simulink model "mux16to1"  (R2020a)
settings: Solver=VariableStepAuto  StartTime=0.0  StopTime=10.0  RelTol=1e-3
settings Model: Creator=kishan  LastModifiedBy=kishan

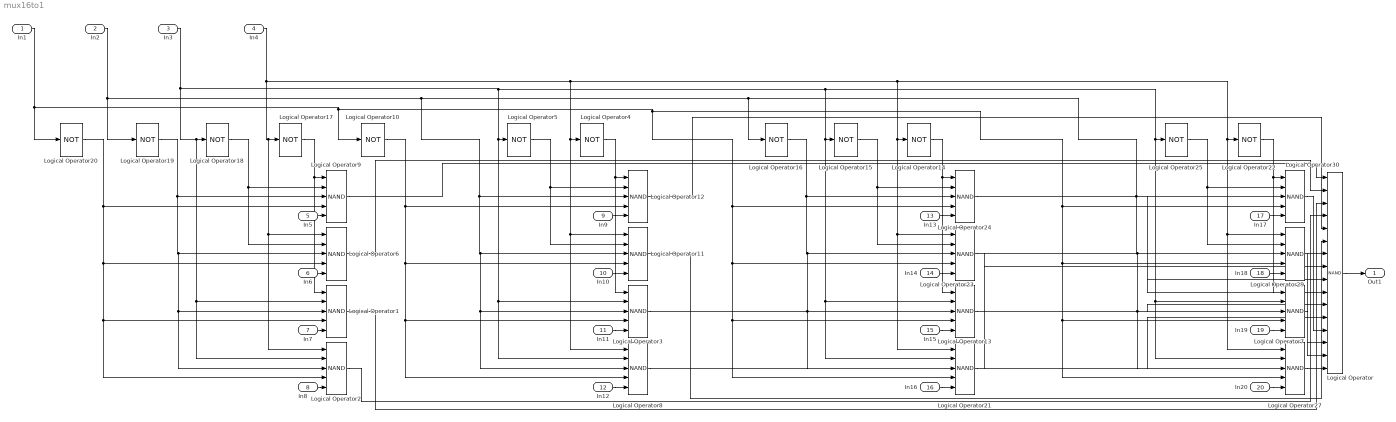
== system mux16to1 ==
  In1 : Inport
  In2 : Inport  Port=2
  In3 : Inport  Port=3
  In4 : Inport  Port=4
  In5 : Inport  Port=5
  In6 : Inport  Port=6
  In7 : Inport  Port=7
  In8 : Inport  Port=8
  In9 : Inport  Port=9
  In10 : Inport  Port=10
  In11 : Inport  Port=11
  In12 : Inport  Port=12
  In13 : Inport  Port=13
  In14 : Inport  Port=14
  In15 : Inport  Port=15
  In16 : Inport  Port=16
  In17 : Inport  Port=17
  In18 : Inport  Port=18
  In19 : Inport  Port=19
  In20 : Inport  Port=20
  Logical Operator : Logic  Operator=NAND  Inputs=16  AllPortsSameDT=off  OutDataTypeStr=boolean
  Logical Operator{1..3,6..9,11..13,21,23..24,27,29..30} (16 alike) : Logic  Operator=NAND  Inputs=5  AllPortsSameDT=off  OutDataTypeStr=boolean
  Logical Operator{4..5,10,14..20,22,25} (12 alike) : Logic  Operator=NOT  AllPortsSameDT=off  OutDataTypeStr=boolean
  Out1 : Outport
  wires:
  Logical Operator17/1 -> Logical Operator1/1, Logical Operator9/1
  Logical Operator18/1 -> Logical Operator6/2, Logical Operator9/2
  Logical Operator19/1 -> Logical Operator2/3, Logical Operator1/3, Logical Operator6/3, Logical Operator9/3
  Logical Operator20/1 -> Logical Operator2/4, Logical Operator1/4, Logical Operator6/4, Logical Operator9/4
  Logical Operator5/1 -> Logical Operator11/2, Logical Operator12/2
  Logical Operator4/1 -> Logical Operator3/1, Logical Operator12/1
  Logical Operator10/1 -> Logical Operator8/4, Logical Operator3/4, Logical Operator11/4, Logical Operator12/4
  Logical Operator15/1 -> Logical Operator23/2, Logical Operator24/2
  Logical Operator16/1 -> Logical Operator21/3, Logical Operator13/3, Logical Operator23/3, Logical Operator24/3
  Logical Operator14/1 -> Logical Operator13/1, Logical Operator24/1
  In4/1 -> Logical Operator27/1, Logical Operator29/1, Logical Operator22/1, Logical Operator21/1, Logical Operator23/1, Logical Operator14/1, Logical Operator8/1, Logical Operator11/1, Logical Operator4/1, Logical Operator2/1, Logical Operator6/1, Logical Operator17/1
  In3/1 -> Logical Operator21/2, Logical Operator13/2, Logical Operator15/1, Logical Operator27/2, Logical Operator7/2, Logical Operator25/1, Logical Operator8/2, Logical Operator3/2, Logical Operator5/1, Logical Operator2/2, Logical Operator1/2, Logical Operator18/1
  Logical Operator25/1 -> Logical Operator29/2, Logical Operator30/2
  In2/1 -> Logical Operator8/3, Logical Operator3/3, Logical Operator11/3, Logical Operator12/3, Logical Operator27/3, Logical Operator7/3, Logical Operator29/3, Logical Operator30/3, Logical Operator16/1, Logical Operator19/1
  Logical Operator22/1 -> Logical Operator7/1, Logical Operator30/1
  In1/1 -> Logical Operator27/4, Logical Operator7/4, Logical Operator29/4, Logical Operator30/4, Logical Operator21/4, Logical Operator13/4, Logical Operator23/4, Logical Operator24/4, Logical Operator10/1, Logical Operator20/1
  Logical Operator9/1 -> Logical Operator/1
  Logical Operator6/1 -> Logical Operator/2
  Logical Operator1/1 -> Logical Operator/3
  Logical Operator2/1 -> Logical Operator/4
  Logical Operator12/1 -> Logical Operator/5
  Logical Operator11/1 -> Logical Operator/6
  Logical Operator3/1 -> Logical Operator/7
  Logical Operator8/1 -> Logical Operator/8
  Logical Operator24/1 -> Logical Operator/9
  Logical Operator23/1 -> Logical Operator/10
  Logical Operator13/1 -> Logical Operator/11
  Logical Operator21/1 -> Logical Operator/12
  Logical Operator30/1 -> Logical Operator/13
  Logical Operator29/1 -> Logical Operator/14
  Logical Operator7/1 -> Logical Operator/15
  Logical Operator27/1 -> Logical Operator/16
  Logical Operator/1 -> Out1/1
  In5/1 -> Logical Operator9/5
  In6/1 -> Logical Operator6/5
  In7/1 -> Logical Operator1/5
  In8/1 -> Logical Operator2/5
  In9/1 -> Logical Operator12/5
  In10/1 -> Logical Operator11/5
  In11/1 -> Logical Operator3/5
  In12/1 -> Logical Operator8/5
  In13/1 -> Logical Operator24/5
  In14/1 -> Logical Operator23/5
  In15/1 -> Logical Operator13/5
  In16/1 -> Logical Operator21/5
  In17/1 -> Logical Operator30/5
  In18/1 -> Logical Operator29/5
  In19/1 -> Logical Operator7/5
  In20/1 -> Logical Operator27/5
